simulink model "Vorletzter_Wert_Signal_bei_Trigger"  (R2013b)
settings: Solver=ode4  StartTime=0.0  StopTime=20  FixedStep=0.01  RelTol=1e-3
settings Model: Creator=daltdoer  LastModifiedBy=daltdoer

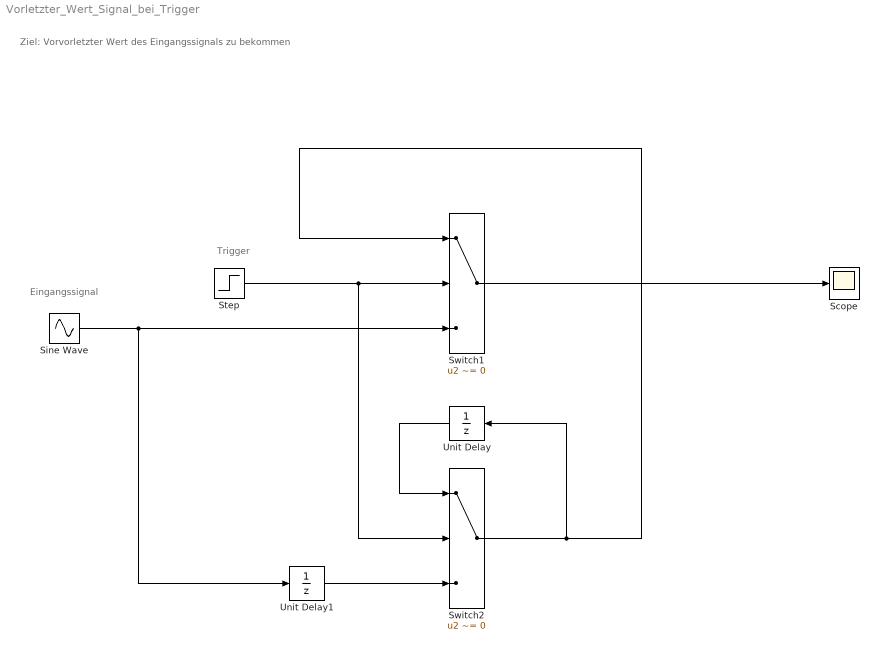
== system Vorletzter_Wert_Signal_bei_Trigger ==
  note: Ziel: Vorvorletzter Wert des Eingangssignals zu bekommen
  note: Trigger
  note: Eingangssignal
  Scope : Scope
  Sine Wave : Sin  SampleTime=0
  Step : Step  Time=5  SampleTime=0
  Switch1 : Switch  Description=#user:ANERTEL#  Criteria=u2 ~= 0  mask(TL_Switch){data={'logdata',{'plotchannels',[]},'output',{'inheritscaling',1},'threshold',{'scalar',1},'autoscaling',{'mode',2},'date',737013.57962427079}}
      settings: CopyFcn=if exist('tl_reset_reviewflag','file')==2,tl_reset_reviewflag(gcbh);end; if exist('block_callbacks') == 2, block_callbacks(gcbh, 'CopyFcn'); end  DeleteFcn=if exist('delete_tlblock','file')==2,delete_tlblock(gcbh);end  NameChangeFcn=if exist('rename_tlblock','file')==2,rename_tlblock(gcbh);end  OpenFcn=if exist('tl_open_blockdlg','file')==2,tl_open_blockdlg(gcbh);else,open_system(gcbh,'parameter');end
      mask Help: eval(['if exist(''tl_online_help'',''file'') == 2, tl_online_help(''Topic'',''TL_Switch''),else, web([''jar:file:///'',matlabroot,''/help/toolbox/simulink/help.jar!/slref/' lower(get_param(gcbh,'Blocktype')) '.html''], ''-helpbrowser''),end'])
      mask Display: plot([-0.05, 1.05, NaN, -0.05, 1.05],[.01, .01, NaN, .99, .99])
  Switch2 : Switch  Description=#user:ANERTEL#  Criteria=u2 ~= 0  mask(TL_Switch){data={'logdata',{'plotchannels',[]},'output',{'inheritscaling',1},'threshold',{'scalar',1},'autoscaling',{'mode',2},'date',737013.5964202662}}
      settings: CopyFcn=if exist('tl_reset_reviewflag','file')==2,tl_reset_reviewflag(gcbh);end; if exist('block_callbacks') == 2, block_callbacks(gcbh, 'CopyFcn'); end  DeleteFcn=if exist('delete_tlblock','file')==2,delete_tlblock(gcbh);end  NameChangeFcn=if exist('rename_tlblock','file')==2,rename_tlblock(gcbh);end  OpenFcn=if exist('tl_open_blockdlg','file')==2,tl_open_blockdlg(gcbh);else,open_system(gcbh,'parameter');end
      mask Help: eval(['if exist(''tl_online_help'',''file'') == 2, tl_online_help(''Topic'',''TL_Switch''),else, web([''jar:file:///'',matlabroot,''/help/toolbox/simulink/help.jar!/slref/' lower(get_param(gcbh,'Blocktype')) '.html''], ''-helpbrowser''),end'])
      mask Display: plot([-0.05, 1.05, NaN, -0.05, 1.05],[.01, .01, NaN, .99, .99])
  Unit Delay : UnitDelay  SampleTime=-1
  Unit Delay1 : UnitDelay  SampleTime=-1
  wires:
  Sine Wave/1 -> Switch1/3, Unit Delay1/1
  Switch1/1 -> Scope/1
  Step/1 -> Switch2/2, Switch1/2
  Unit Delay1/1 -> Switch2/3
  Switch2/1 -> Unit Delay/1, Switch1/1
  Unit Delay/1 -> Switch2/1
